simulink model "Antriebe_P_Var"  (Simulink 7.6)
settings: Solver=ode45  StartTime=0.0  StopTime=SimulTime  RelTol=1e-3
values from neighbouring files (symbols this model uses):
  Ein = 1    [ParamtersAntriebe_P_Var.m]
  hsp = 200    [ParamtersAntriebe_P_Var.m]
  m = 15    [ParamtersAntriebe_P_Var.m]
  MaxDrehmoment = 38    [ParamtersAntriebe_P_Var.m]
  MaxDrehzahl = 3000    [ParamtersAntriebe_P_Var.m]
  PR = 25    [ParamtersAntriebe_P_Var.m]
  r = 0.2    [ParamtersAntriebe_P_Var.m]
undefined symbols (not defined in the file or in its folder): Antriebe, Job
settings Model: Creator=Coni  LastModifiedBy=conid

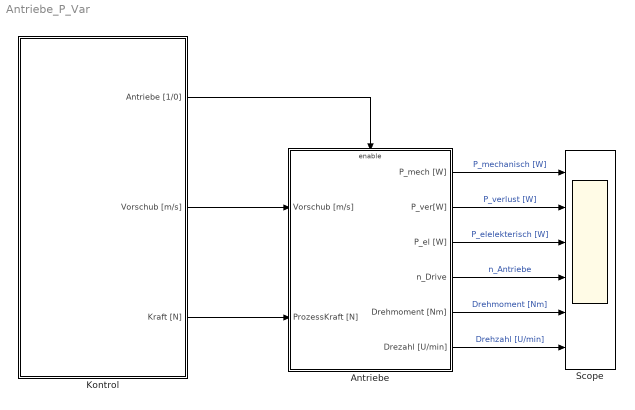
== system Antriebe_P_Var ==
  Antriebe : Subsystem  TreatAsAtomicUnit=on
  Kontrol : Subsystem  TreatAsAtomicUnit=on  mask{Antriebe=[0 1 1 1 1], Job=Job}
      mask prompts: Job "Job Struct"
      mask help:
      | Controls the components of the machine:
      |
      | Status:
      |     0. Off
      |     1. Standby
      |     2. Warmup
      |     3. Setting
      |     4. Machining
      |
      | If the status is machining, the job defined as
      |     - Job.time
      |     - Job.omega_dem
      |     - Job.M_dem
      | will be runned, and repeated.
      mask TabNameString: Status,Job
  Scope : Scope  NumInputPorts=6
      settings: TickLabels=on  TimeRange=2  YMin=0.014~0.036~0.022~0.3705~-5~-5  YMax=0.01575~0.0405~0.0245~0.4095~5~5  SaveName=Scp_Drives
  wires:
  Antriebe/1(P_mech [W]) -> Scope/1  "P_mechanisch [W]"
  Antriebe/2(P_ver[W]) -> Scope/2  "P_verlust [W]"
  Antriebe/3(P_el [W]) -> Scope/3  "P_elelekterisch [W]"
  Antriebe/4(n_Drive) -> Scope/4  "n_Antriebe"
  Kontrol/1(Antriebe [1/0]) -> Antriebe/Enable
  Kontrol/2(Vorschub [m/s]) -> Antriebe/1(Vorschub [m/s])
  Kontrol/3(Kraft [N]) -> Antriebe/2(ProzessKraft [N])
  Antriebe/5(Drehmoment [Nm]) -> Scope/5  "Drehmoment [Nm]"
  Antriebe/6(Drezahl [U/min]) -> Scope/6  "Drehzahl [U/min]"

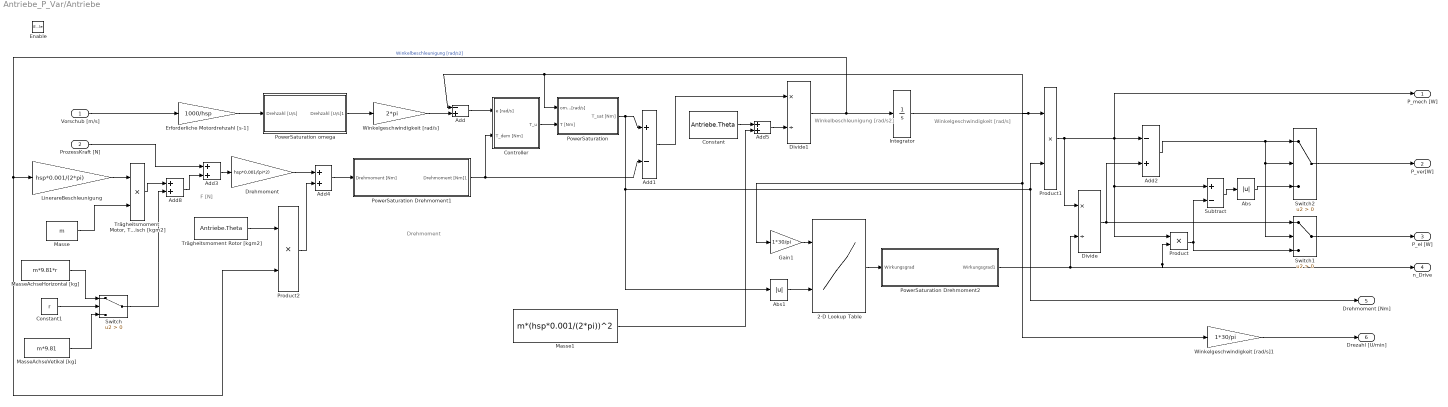
== system Antriebe_P_Var/Antriebe ==
  note: Winkelgeschwindigkeit [rad/s]
  note: Drehmoment
  note: F [N]
  note: Winkelbeschleunigung [rad/s2]
  Vorschub [m/s] : Inport
  ProzessKraft [N] : Inport  Port=2
  Enable : EnablePort
  2-D Lookup Table : Lookup_n-D  BreakpointsForDimension1=Antriebe.Tabelomega  BreakpointsForDimension2=Antriebe.TabelM  BreakpointsForDimension1Min=[0]  BreakpointsForDimension2Min=[0]  BreakpointsForDimension1Max=[3000]  BreakpointsForDimension2Max=[9.5]  Table=Antriebe.Tabeleta  TableMin=[0]  TableMax=[1]  InterpMethod=Cubic spline  OutMin=[0]  OutMax=[1]  RndMeth=Simplest  InputSameDT=on
  Abs : Abs
  Abs1 : Abs
  Add : Sum  Inputs=-+
  Add1 : Sum  Inputs=+-
  Add2 : Sum  Inputs=-+
  Add{3..5,8} (4 alike) : Sum
  Constant : Constant  Value=Antriebe.Theta
  Constant1 : Constant  Value=r
  Controller : Subsystem  TreatAsAtomicUnit=on
  Divide : Product  Inputs=*/
  Divide1 : Product  Inputs=*/
  Drehmoment : Gain  Gain=hsp*0.001/(pi*2)
  Erforderliche Motordrehzahl [s-1] : Gain  Gain=1000/hsp
  Gain1 : Gain  Gain=1*30/pi
  Integrator : Integrator
  LinerareBeschleunigung : Gain  Gain=hsp*0.001/(2*pi)
  Masse : Constant  Value=m
  Masse1 : Constant  Value=m*(hsp*0.001/(2*pi))^2
  MasseAchseHorizontal [kg] : Constant  Value=m*9.81*r
  MasseAchseVetikal [kg] : Constant  Value=m*9.81
  PowerSaturation : Subsystem  TreatAsAtomicUnit=on
  PowerSaturation Drehmoment1 : Subsystem  TreatAsAtomicUnit=on
  PowerSaturation Drehmoment2 : Subsystem  TreatAsAtomicUnit=on
  PowerSaturation omega : Subsystem  TreatAsAtomicUnit=on
  Product : Product  RndMeth=Zero
  Product1 : Product  RndMeth=Zero
  Product2 : Product  RndMeth=Zero
  Subtract : Sum  Inputs=+-
  Switch : Switch  Criteria=u2 > Threshold
  Switch1 : Switch  Criteria=u2 > Threshold
  Switch2 : Switch  Criteria=u2 > Threshold
  "Trägheitsmoment  Motor, Tisch [kgm2]" : Product  RndMeth=Zero
  Trägheitsmoment Rotor [kgm2] : Constant  Value=Antriebe.Theta
  Winkelgeschwindigkeit [rad/s] : Gain  Gain=2*pi
  Winkelgeschwindigkeit [rad/s]1 : Gain  Gain=1*30/pi
  P_mech [W] : Outport
  P_ver[W] : Outport  Port=2
  P_el [W] : Outport  Port=3
  n_Drive : Outport  Port=4
  Drehmoment [Nm] : Outport  Port=5
  Drezahl [U/min] : Outport  Port=6
  wires:
  Add/1 -> Controller/1(e [rad/s])
  Controller/1(T_u) -> PowerSaturation/2(T [Nm])
  PowerSaturation/1(T_sat [Nm]) -> Add1/1, Abs1/1, Product1/2, Drehmoment [Nm]/1
  Divide1/1 -> Integrator/1, LinerareBeschleunigung/1, Product2/2  "Winkelbeschleunigung [rad/s2]"
  Integrator/1 -> Add/1, PowerSaturation/1(omega [rad/s]), Product1/1, Gain1/1, Winkelgeschwindigkeit [rad/s]1/1
  Product1/1 -> Divide/1, P_mech [W]/1, Add2/1, Subtract/1, Product/1
  Divide/1 -> Add2/2, Switch1/1
  Gain1/1 -> 2-D Lookup Table/1
  Add1/1 -> Divide1/1
  Add3/1 -> Drehmoment/1
  ProzessKraft [N]/1 -> Add3/1
  Add5/1 -> Divide1/2
  Constant/1 -> Add5/1
  Trägheitsmoment Rotor [kgm2]/1 -> Product2/1
  Product2/1 -> Add4/2
  MasseAchseHorizontal [kg]/1 -> Switch/1
  MasseAchseVetikal [kg]/1 -> Switch/3
  Constant1/1 -> Switch/2
  Vorschub [m/s]/1 -> Erforderliche Motordrehzahl [s-1]/1
  Masse1/1 -> Add5/2
  Add8/1 -> Add3/2
  Switch/1 -> Add8/2
  Masse/1 -> "Trägheitsmoment  Motor, Tisch [kgm2]"/2
  "Trägheitsmoment  Motor, Tisch [kgm2]"/1 -> Add8/1
  LinerareBeschleunigung/1 -> "Trägheitsmoment  Motor, Tisch [kgm2]"/1
  Winkelgeschwindigkeit [rad/s]/1 -> Add/2
  PowerSaturation omega/1(Drehzahl [U/s]1) -> Winkelgeschwindigkeit [rad/s]/1
  Erforderliche Motordrehzahl [s-1]/1 -> PowerSaturation omega/1(Drehzahl [U/s])
  Add2/1 -> Switch2/1, Switch2/2, Switch1/2
  Product/1 -> Subtract/2, Switch1/3
  Subtract/1 -> Abs/1
  Abs/1 -> Switch2/3
  Switch2/1 -> P_ver[W]/1
  Switch1/1 -> P_el [W]/1
  Abs1/1 -> 2-D Lookup Table/2
  Winkelgeschwindigkeit [rad/s]1/1 -> Drezahl [U/min]/1
  Drehmoment/1 -> Add4/1
  Add4/1 -> PowerSaturation Drehmoment1/1(Drehmoment [Nm])
  PowerSaturation Drehmoment1/1(Drehmoment [Nm]1) -> Add1/2, Controller/2(T_dem [Nm])
  2-D Lookup Table/1 -> PowerSaturation Drehmoment2/1(Wirkungsgrad)
  PowerSaturation Drehmoment2/1(Wirkungsgrad1) -> Divide/2, Product/2, n_Drive/1

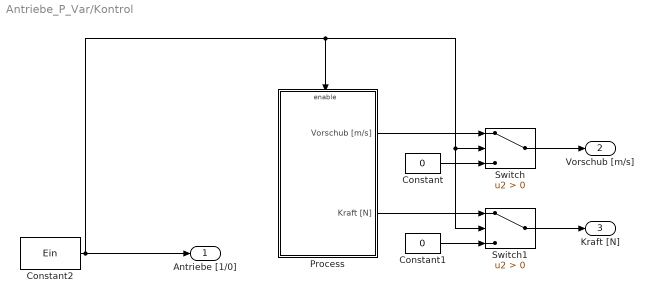
== system Antriebe_P_Var/Kontrol ==
  Constant : Constant  Value=0
  Constant1 : Constant  Value=0
  Constant2 : Constant  Value=Ein
  Process : Subsystem  TreatAsAtomicUnit=on
  Switch : Switch  Criteria=u2 > Threshold
  Switch1 : Switch  Criteria=u2 > Threshold
  Antriebe [1/0] : Outport
  Vorschub [m/s] : Outport  Port=2
  Kraft [N] : Outport  Port=3
  wires:
  Constant2/1 -> Process/Enable, Switch1/2, Switch/2, Antriebe [1/0]/1
  Process/1(Vorschub [m/s]) -> Switch/1
  Constant/1 -> Switch/3
  Process/2(Kraft [N]) -> Switch1/1
  Constant1/1 -> Switch1/3
  Switch/1 -> Vorschub [m/s]/1
  Switch1/1 -> Kraft [N]/1

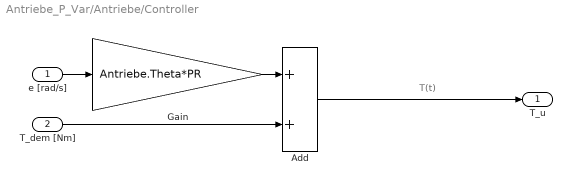
== system Antriebe_P_Var/Antriebe/Controller ==
  note: T(t)
  e [rad/s] : Inport
  T_dem [Nm] : Inport  Port=2
  Add : Sum
  Gain : Gain  Gain=Antriebe.Theta*PR
  T_u : Outport
  wires:
  Add/1 -> T_u/1
  T_dem [Nm]/1 -> Add/2
  Gain/1 -> Add/1
  e [rad/s]/1 -> Gain/1

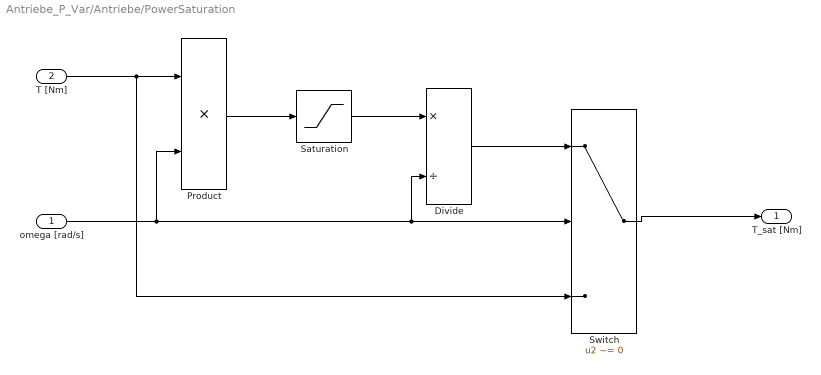
== system Antriebe_P_Var/Antriebe/PowerSaturation ==
  omega [rad/s] : Inport
  T [Nm] : Inport  Port=2
  Divide : Product  Inputs=*/
  Product : Product  RndMeth=Zero
  Saturation : Saturate  UpperLimit=Antriebe.Pmax  LowerLimit=-Antriebe.Pmax  ZeroCross=off
  Switch : Switch  Criteria=u2 ~= 0
  T_sat [Nm] : Outport
  wires:
  Product/1 -> Saturation/1
  Saturation/1 -> Divide/1
  Divide/1 -> Switch/1
  Switch/1 -> T_sat [Nm]/1
  T [Nm]/1 -> Product/1, Switch/3
  omega [rad/s]/1 -> Switch/2, Divide/2, Product/2

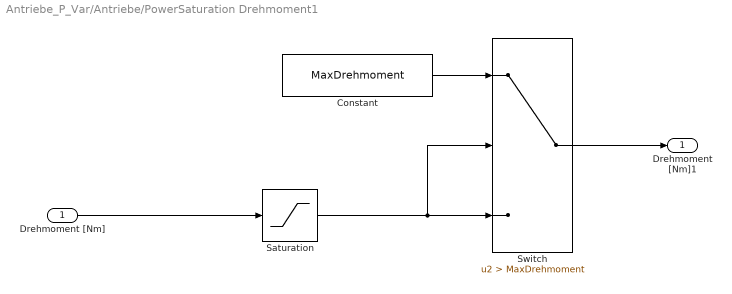
== system Antriebe_P_Var/Antriebe/PowerSaturation Drehmoment1 ==
  Drehmoment [Nm] : Inport
  Constant : Constant  Value=MaxDrehmoment
  Saturation : Saturate  UpperLimit=MaxDrehmoment  LowerLimit=-MaxDrehmoment  ZeroCross=off
  Switch : Switch  Criteria=u2 > Threshold  Threshold=MaxDrehmoment
  Drehmoment [Nm]1 : Outport
  wires:
  Saturation/1 -> Switch/3, Switch/2
  Constant/1 -> Switch/1
  Drehmoment [Nm]/1 -> Saturation/1
  Switch/1 -> Drehmoment [Nm]1/1

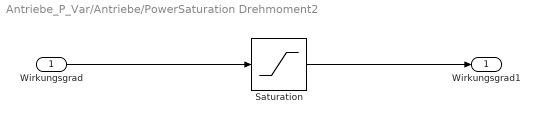
== system Antriebe_P_Var/Antriebe/PowerSaturation Drehmoment2 ==
  Wirkungsgrad : Inport
  Saturation : Saturate  UpperLimit=0.95  LowerLimit=0.1  ZeroCross=off
  Wirkungsgrad1 : Outport
  wires:
  Wirkungsgrad/1 -> Saturation/1
  Saturation/1 -> Wirkungsgrad1/1

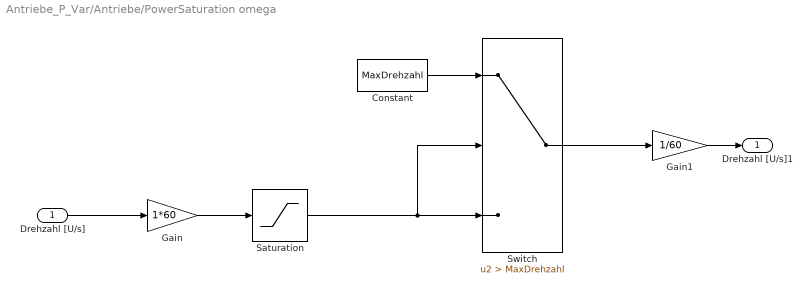
== system Antriebe_P_Var/Antriebe/PowerSaturation omega ==
  Drehzahl [U/s] : Inport
  Constant : Constant  Value=MaxDrehzahl
  Gain : Gain  Gain=1*60
  Gain1 : Gain  Gain=1/60
  Saturation : Saturate  UpperLimit=MaxDrehzahl  LowerLimit=0  ZeroCross=off
  Switch : Switch  Criteria=u2 > Threshold  Threshold=MaxDrehzahl
  Drehzahl [U/s]1 : Outport
  wires:
  Saturation/1 -> Switch/3, Switch/2
  Constant/1 -> Switch/1
  Drehzahl [U/s]/1 -> Gain/1
  Gain/1 -> Saturation/1
  Gain1/1 -> Drehzahl [U/s]1/1
  Switch/1 -> Gain1/1

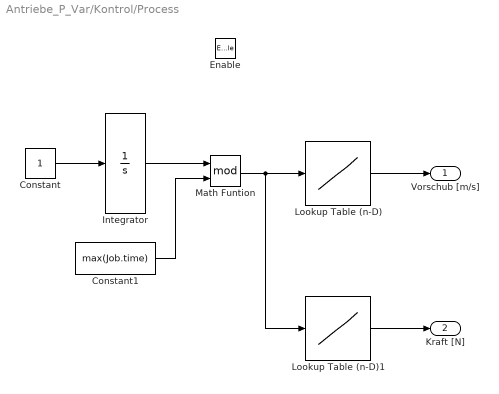
== system Antriebe_P_Var/Kontrol/Process ==
  Enable : EnablePort
  Constant : Constant
  Constant1 : Constant  Value=max(Job.time)
  Integrator : Integrator
  Lookup Table (n-D) : Lookup_n-D  NumberOfTableDimensions=1  BreakpointsForDimension1=Job.time  Table=Job.Vorschub  InterpMethod=None - Flat  ExtrapMethod=Cubic spline  InputSameDT=on
  Lookup Table (n-D)1 : Lookup_n-D  NumberOfTableDimensions=1  BreakpointsForDimension1=Job.time  Table=Job.Kraft  InterpMethod=None - Flat  ExtrapMethod=Cubic spline  InputSameDT=on
  Math Funtion : Math  Operator=mod  SaturateOnIntegerOverflow=on
  Vorschub [m/s] : Outport
  Kraft [N] : Outport  Port=2
  wires:
  Constant/1 -> Integrator/1
  Integrator/1 -> Math Funtion/1
  Math Funtion/1 -> Lookup Table (n-D)/1, Lookup Table (n-D)1/1
  Lookup Table (n-D)/1 -> Vorschub [m/s]/1
  Lookup Table (n-D)1/1 -> Kraft [N]/1
  Constant1/1 -> Math Funtion/2
